simulink model "nonlinearwithoutcontroller"  (R2016a)
settings: Solver=VariableStepAuto  StartTime=0.0  StopTime=10000  RelTol=1e-3
settings Model: Creator=ASUS  LastModifiedBy=ASUS

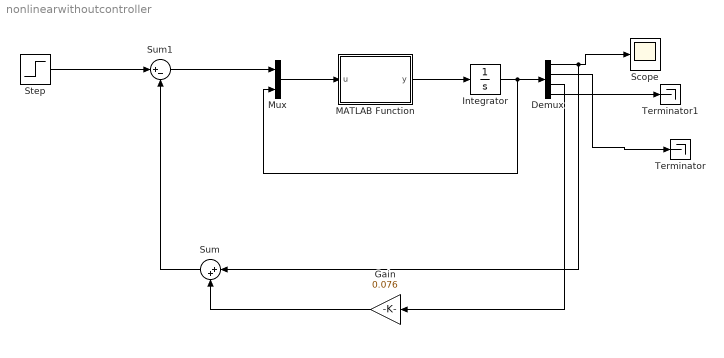
== system nonlinearwithoutcontroller ==
  Demux : Demux
  Gain : Gain  Gain=0.076
  Integrator : Integrator
  MATLAB Function : MATLAB Function  TreatAsAtomicUnit=on
  Mux : Mux  Inputs=2
  Scope : Scope
  Step : Step  SampleTime=0
  Sum : Sum  Inputs=|++
  Sum1 : Sum  Inputs=|+-
  Terminator : Terminator
  Terminator1 : Terminator
  wires:
  MATLAB Function/1(y) -> Integrator/1
  Mux/1 -> MATLAB Function/1(u)
  Integrator/1 -> Demux/1, Mux/2
  Demux/1 -> Sum/1, Scope/1
  Demux/2 -> Terminator/1
  Demux/3 -> Gain/1
  Gain/1 -> Sum/2
  Demux/4 -> Terminator1/1
  Sum/1 -> Sum1/2
  Step/1 -> Sum1/1
  Sum1/1 -> Mux/1

== matlab function nonlinearwithoutcontroller/MATLAB Function ==
  data: u input; y output
function y = fcn(u)
%#codegen
c1 = 1350;
c2 = 1350/4;
c3 = 1350/2;
c4 = 2700;
c5 = 1350;
c6 = 3091;
a = 0.734;
b = 0.67391;
w = 18;
uu = u(1);
x = u(2:5);
y = u(1:4);
y(1) = x(2);
y(2) = (-8*c1^2*x(2)*x(3)*x(4)+(c5*a+b*c4)*(-2*c1*x(2)^2*x(3)+2*c1*x(3)*w^2) + 2*c1*uu)/(2*c1*c6+4*c1^2*x(3)^2-c5^2*a^2-2*c5*a*c4*b-c4^2*b^2);
y(3) = x(4);
y(4) = (4*(c5*a+c4*b)*c1*x(2)*x(3)*x(4)-(c6+2*c1*x(3)^2)*(-2*c1*x(2)^2*x(3)+2*c1*x(3)*w^2)-(c5*a+c4*b)*uu)/(2*c1*c6+4*c1^2*x(3)^2-c5^2*a^2-2*c5*a*c4*b-c4^2*b^2);
